simulink model "aerotest"  (R2021b)
settings: Solver=VariableStepAuto  StartTime=0.0  StopTime=10.0  RelTol=1e-3
undefined symbols (not defined in the file or in its folder): admireDB
libraries: simulink_extras x103, simulink x24, aerolibatmos2 x1
(part 5 of 13)

== system aerotest/RollMomentCoefficient/MachRegion1/Crmbetad ==
  in_bus : Inport
  Bus Selector : BusSelector  OutputSignals=AeroIn_Bus.angleOfAttack_deg,AeroIn_Bus.betad
  Crmbetad_ : Subsystem
  Crmbetad : Outport
  wires:
  Bus Selector/1 -> Crmbetad_/1(angleOfAttack_deg)  "<angleOfAttack_deg>"
  Bus Selector/2 -> Crmbetad_/2(betad)  "<betad>"
  in_bus/1 -> Bus Selector/1  "in_bus"
  Crmbetad_/1(Crmbetad) -> Crmbetad/1

== system aerotest/RollMomentCoefficient/MachRegion1/Crmblg ==
  in_bus : Inport
  Bus Selector : BusSelector  OutputSignals=AeroIn_Bus.lg_bool,AeroIn_Bus.angleOfAttack_deg,AeroIn_Bus.angleOfSideslip_deg
  Crmblg_ : Subsystem
  Crmblg : Outport
  wires:
  Bus Selector/3 -> Crmblg_/3(angleOfSideslip_deg)  "<angleOfSideslip_deg>"
  Bus Selector/2 -> Crmblg_/2(angleOfAttack_deg)  "<angleOfAttack_deg>"
  Bus Selector/1 -> Crmblg_/1(dLG)  "<lg_bool>"
  in_bus/1 -> Bus Selector/1  "in_bus"
  Crmblg_/1(Crmblg) -> Crmblg/1

== system aerotest/RollMomentCoefficient/MachRegion1/Crmdai ==
  in_bus : Inport
  Bus Selector : BusSelector  OutputSignals=AeroIn_Bus.dAI,AeroIn_Bus.angleOfAttack_deg,AeroIn_Bus.dEI,eieff,AeroIn_Bus.qacorr,AeroIn_Bus.mach_nd
  Crmdai_ : Subsystem
  Crmdai : Outport
  wires:
  Bus Selector/1 -> Crmdai_/1(dAI)  "<dAI>"
  Bus Selector/2 -> Crmdai_/2(angleOfAttack_deg)  "<angleOfAttack_deg>"
  Bus Selector/3 -> Crmdai_/3(dEI)  "<dEI>"
  Bus Selector/4 -> Crmdai_/4(eieff)  "<eieff>"
  Bus Selector/5 -> Crmdai_/5(qacorr)  "<qacorr>"
  Bus Selector/6 -> Crmdai_/6(mach_nd)  "<mach_nd>"
  in_bus/1 -> Bus Selector/1  "in_bus"
  Crmdai_/1(Crmdai) -> Crmdai/1

== system aerotest/RollMomentCoefficient/MachRegion1/Crmdaib ==
  in_bus : Inport
  Bus Selector : BusSelector  OutputSignals=AeroIn_Bus.angleOfAttack_deg,AeroIn_Bus.dAI,AeroIn_Bus.angleOfSideslip_deg,eieff
  Crmdaib_ : Subsystem
  Crmdaib : Outport
  wires:
  Bus Selector/1 -> Crmdaib_/1(angleOfAttack_deg)  "<angleOfAttack_deg>"
  Bus Selector/2 -> Crmdaib_/2(dAI)  "<dAI>"
  Bus Selector/3 -> Crmdaib_/3(angleOfSideslip_deg)  "<angleOfSideslip_deg>"
  Bus Selector/4 -> Crmdaib_/4(eieff)  "<eieff>"
  Crmdaib_/1(Crmdaib) -> Crmdaib/1
  in_bus/1 -> Bus Selector/1  "in_bus"

== system aerotest/RollMomentCoefficient/MachRegion1/Crmday ==
  in_bus : Inport
  Bus Selector : BusSelector  OutputSignals=AeroIn_Bus.dAY,AeroIn_Bus.angleOfAttack_deg,AeroIn_Bus.dEY,eoeff,AeroIn_Bus.qacorr,AeroIn_Bus.mach_nd
  Crmday_ : Subsystem
  Crmday : Outport
  wires:
  Crmday_/1(Crmdai) -> Crmday/1
  in_bus/1 -> Bus Selector/1  "in_bus"
  Bus Selector/6 -> Crmday_/6(mach_nd)  "<mach_nd>"
  Bus Selector/5 -> Crmday_/5(qacorr)  "<qacorr>"
  Bus Selector/4 -> Crmday_/4(eoeff)  "<eoeff>"
  Bus Selector/3 -> Crmday_/3(dEY)  "<dEY>"
  Bus Selector/2 -> Crmday_/2(angleOfAttack_deg)  "<angleOfAttack_deg>"
  Bus Selector/1 -> Crmday_/1(dAY)  "<dAY>"

== system aerotest/RollMomentCoefficient/MachRegion1/Crmdayb ==
  in_bus : Inport
  Bus Selector : BusSelector  OutputSignals=AeroIn_Bus.angleOfAttack_deg,AeroIn_Bus.dAY,AeroIn_Bus.angleOfSideslip_deg,eoeff
  Crmdaib_ : Subsystem
  Crmdayb : Outport
  wires:
  in_bus/1 -> Bus Selector/1  "in_bus"
  Crmdaib_/1(Crmdaib) -> Crmdayb/1
  Bus Selector/4 -> Crmdaib_/4(eoeff)  "<eoeff>"
  Bus Selector/3 -> Crmdaib_/3(angleOfSideslip_deg)  "<angleOfSideslip_deg>"
  Bus Selector/2 -> Crmdaib_/2(dAY)  "<dAY>"
  Bus Selector/1 -> Crmdaib_/1(angleOfAttack_deg)  "<angleOfAttack_deg>"

== system aerotest/RollMomentCoefficient/MachRegion1/Crmdna ==
  in_bus : Inport
  Bus Selector : BusSelector  OutputSignals=AeroIn_Bus.dNE,AeroIn_Bus.angleOfAttack_deg,AeroIn_Bus.dNA
  Crmdna_ : Subsystem
  Crmdna : Outport
  wires:
  Bus Selector/3 -> Crmdna_/3(dNA)  "<dNA>"
  Bus Selector/2 -> Crmdna_/2(angleOfAttack_deg)  "<angleOfAttack_deg>"
  Bus Selector/1 -> Crmdna_/1(dNE)  "<dNE>"
  Crmdna_/1(Crmdna) -> Crmdna/1
  in_bus/1 -> Bus Selector/1  "in_bus"

== system aerotest/RollMomentCoefficient/MachRegion1/Crmdr ==
  in_bus : Inport
  Bus Selector : BusSelector  OutputSignals=AeroIn_Bus.angleOfAttack_deg,AeroIn_Bus.rud_deg,AeroIn_Bus.angleOfSideslip_deg,AeroIn_Bus.qacorr,AeroIn_Bus.mach_nd
  Crmdr_ : Subsystem
  Crmdr : Outport
  wires:
  Bus Selector/5 -> Crmdr_/5(mach_nd)  "<mach_nd>"
  Bus Selector/4 -> Crmdr_/4(qacorr)  "<qacorr>"
  Bus Selector/3 -> Crmdr_/3(angleOfSideslip_deg)  "<angleOfSideslip_deg>"
  Bus Selector/2 -> Crmdr_/2(dR)  "<rud_deg>"
  Bus Selector/1 -> Crmdr_/1(angleOfAttack_deg)  "<angleOfAttack_deg>"
  Crmdr_/1(Crmdr) -> Crmdr/1
  in_bus/1 -> Bus Selector/1  "in_bus"

== system aerotest/RollMomentCoefficient/MachRegion1/Crmp ==
  in_bus : Inport
  Bus Selector : BusSelector  OutputSignals=AeroIn_Bus.dN,AeroIn_Bus.angleOfAttack_deg,AeroIn_Bus.qacorr,AeroIn_Bus.mach_nd,AeroIn_Bus.pc
  Crmp_ : Subsystem
  Crmp : Outport
  wires:
  Bus Selector/1 -> Crmp_/1(dN)  "<dN>"
  Bus Selector/2 -> Crmp_/2(angleOfAttack_deg)  "<angleOfAttack_deg>"
  Bus Selector/3 -> Crmp_/3(qacorr)  "<qacorr>"
  Bus Selector/4 -> Crmp_/4(mach_nd)  "<mach_nd>"
  Bus Selector/5 -> Crmp_/5(pc)  "<pc>"
  Crmp_/1(Crmp) -> Crmp/1
  in_bus/1 -> Bus Selector/1  "in_bus"

== system aerotest/RollMomentCoefficient/MachRegion1/Crmpbeta ==
  in_bus : Inport
  Bus Selector : BusSelector  OutputSignals=AeroIn_Bus.angleOfSideslip_deg,AeroIn_Bus.angleOfAttack_deg,AeroIn_Bus.pc
  Crmpbeta_ : Subsystem
  Crmpbeta : Outport
  wires:
  Bus Selector/1 -> Crmpbeta_/1(angleOfSideslip_deg)  "<angleOfSideslip_deg>"
  Bus Selector/2 -> Crmpbeta_/2(angleOfAttack_deg)  "<angleOfAttack_deg>"
  Bus Selector/3 -> Crmpbeta_/3(pc)  "<pc>"
  in_bus/1 -> Bus Selector/1  "in_bus"
  Crmpbeta_/1(Crmpbeta) -> Crmpbeta/1

== system aerotest/RollMomentCoefficient/MachRegion1/Crmr ==
  in_bus : Inport
  Bus Selector : BusSelector  OutputSignals=AeroIn_Bus.dN,AeroIn_Bus.angleOfAttack_deg,AeroIn_Bus.rc
  Crmr_ : Subsystem
  Crmr : Outport
  wires:
  Bus Selector/1 -> Crmr_/1(dN)  "<dN>"
  Bus Selector/2 -> Crmr_/2(angleOfAttack_deg)  "<angleOfAttack_deg>"
  Bus Selector/3 -> Crmr_/3(rc)  "<rc>"
  Crmr_/1(Crmr) -> Crmr/1
  in_bus/1 -> Bus Selector/1  "in_bus"

== system aerotest/RollMomentCoefficient/MachRegion1/Crmrbeta ==
  in_bus : Inport
  Bus Selector : BusSelector  OutputSignals=AeroIn_Bus.angleOfSideslip_deg,AeroIn_Bus.angleOfAttack_deg,AeroIn_Bus.rc
  Crmrbeta_ : Subsystem
  Crmrbeta : Outport
  wires:
  in_bus/1 -> Bus Selector/1  "in_bus"
  Crmrbeta_/1(Crmrbeta) -> Crmrbeta/1
  Bus Selector/3 -> Crmrbeta_/3(rc)  "<rc>"
  Bus Selector/2 -> Crmrbeta_/2(angleOfAttack_deg)  "<angleOfAttack_deg>"
  Bus Selector/1 -> Crmrbeta_/1(angleOfSideslip_deg)  "<angleOfSideslip_deg>"

== system aerotest/RollMomentCoefficient/MachRegion1/Crmrde ==
  in_bus : Inport
  Bus Selector : BusSelector  OutputSignals=AeroIn_Bus.mach_nd,AeroIn_Bus.angleOfAttack_deg,AeroIn_Bus.rc,AeroIn_Bus.dEI,eieff,AeroIn_Bus.dEY,eoeff
  Crmrde_ : Subsystem
  Crmrbeta : Outport
  wires:
  Bus Selector/1 -> Crmrde_/1(mach_nd)  "<mach_nd>"
  Bus Selector/2 -> Crmrde_/2(angleOfAttack_deg)  "<angleOfAttack_deg>"
  Bus Selector/3 -> Crmrde_/3(rc)  "<rc>"
  Bus Selector/4 -> Crmrde_/4(dEI)  "<dEI>"
  Bus Selector/5 -> Crmrde_/5(eieff)  "<eieff>"
  Bus Selector/6 -> Crmrde_/6(dey)  "<dEY>"
  Bus Selector/7 -> Crmrde_/7(eoeff)  "<eoeff>"
  Crmrde_/1(Crmrbeta) -> Crmrbeta/1
  in_bus/1 -> Bus Selector/1  "in_bus"

== system aerotest/RollMomentCoefficient/MachRegion1/eoeff1 ==
  AeroIn_Bus : Inport
  Bus Selector : BusSelector  OutputSignals=mach_nd
  CRMDAYOD_M : Lookup_n-D  NumberOfTableDimensions=1  BreakpointsForDimension1=admireDB.aerodata_asym_ext.CRMDAYOD.breakpoints.M  BreakpointsForDimension3=[5, 7]  Table=admireDB.aerodata_asym_ext.CRMDAYOD.newTable  ExtrapMethod=Clip  InternalRulePriority=Speed  RndMeth=Simplest  InputSameDT=on
  Constant : Constant
  Sum : Sum  Inputs=-+|
  eoeff : Outport
  eieff : Outport  Port=2
  wires:
  Sum/1 -> eieff/1
  CRMDAYOD_M/1 -> eoeff/1, Sum/1
  Constant/1 -> Sum/2
  Bus Selector/1 -> CRMDAYOD_M/1  "<mach_nd>"
  AeroIn_Bus/1 -> Bus Selector/1

== system aerotest/RollMomentCoefficient/MachRegion2/Crmbasic ==
  in_bus : Inport
  Bus Selector : BusSelector  OutputSignals=AeroIn_Bus.angleOfAttack_deg,AeroIn_Bus.tflow
  Crmbasic_ : Subsystem
  Crmbasic : Outport
  wires:
  Bus Selector/2 -> Crmbasic_/2(tflow)  "<tflow>"
  Crmbasic_/1(Crmbasic) -> Crmbasic/1
  Bus Selector/1 -> Crmbasic_/1(angleOfAttack_deg)  "<angleOfAttack_deg>"
  in_bus/1 -> Bus Selector/1  "in_bus"

== system aerotest/RollMomentCoefficient/MachRegion2/Crmbde ==
  in_bus : Inport
  Bus Selector : BusSelector  OutputSignals=AeroIn_Bus.angleOfAttack_deg,AeroIn_Bus.dN,AeroIn_Bus.dEI,AeroIn_Bus.angleOfSideslip_deg,AeroIn_Bus.dEY,eieff,eoeff
  Crmbde_ : Subsystem
  Crmbde : Outport
  wires:
  Bus Selector/1 -> Crmbde_/1(angleOfAttack_deg)  "<angleOfAttack_deg>"
  Bus Selector/2 -> Crmbde_/2(dN)  "<dN>"
  Bus Selector/3 -> Crmbde_/3(dEI)  "<dEI>"
  Bus Selector/4 -> Crmbde_/4(angleOfSideslip_deg)  "<angleOfSideslip_deg>"
  Bus Selector/5 -> Crmbde_/5(dEY)  "<dEY>"
  Bus Selector/6 -> Crmbde_/6(eieff)  "<eieff>"
  Bus Selector/7 -> Crmbde_/7(eoeff)  "<eoeff>"
  Crmbde_/1(Crmbde) -> Crmbde/1
  in_bus/1 -> Bus Selector/1  "in_bus"

== system aerotest/RollMomentCoefficient/MachRegion2/Crmbdle ==
  in_bus : Inport
  Bus Selector : BusSelector  OutputSignals=AeroIn_Bus.angleOfAttack_deg,AeroIn_Bus.dEI,AeroIn_Bus.angleOfSideslip_deg,AeroIn_Bus.lef_deg,AeroIn_Bus.dEY,AeroIn_Bus.tflow,AeroIn_Bus.tfhigh
  Crmbdle_ : Subsystem
  Crmbdle : Outport
  wires:
  Bus Selector/7 -> Crmbdle_/7(tfhigh)  "<tfhigh>"
  Bus Selector/6 -> Crmbdle_/6(tflow)  "<tflow>"
  Bus Selector/5 -> Crmbdle_/5(dEY)  "<dEY>"
  Bus Selector/4 -> Crmbdle_/4(dLE)  "<lef_deg>"
  Bus Selector/3 -> Crmbdle_/3(angleOfSideslip_deg)  "<angleOfSideslip_deg>"
  Bus Selector/2 -> Crmbdle_/2(dEI)  "<dEI>"
  Bus Selector/1 -> Crmbdle_/1(angleOfAttack_deg)  "<angleOfAttack_deg>"
  Crmbdle_/1(Crmbdle) -> Crmbdle/1
  in_bus/1 -> Bus Selector/1  "in_bus"

== system aerotest/RollMomentCoefficient/MachRegion2/Crmbdn ==
  in_bus : Inport
  Bus Selector : BusSelector  OutputSignals=AeroIn_Bus.angleOfSideslip_deg,AeroIn_Bus.dN,AeroIn_Bus.angleOfAttack_deg,AeroIn_Bus.tflow,AeroIn_Bus.tfhigh
  Crmbdn_ : Subsystem
  Crmbdn : Outport
  wires:
  Bus Selector/1 -> Crmbdn_/1(angleOfSideslip_deg)  "<angleOfSideslip_deg>"
  Bus Selector/2 -> Crmbdn_/2(dN)  "<dN>"
  Bus Selector/3 -> Crmbdn_/3(angleOfAttack_deg)  "<angleOfAttack_deg>"
  Bus Selector/4 -> Crmbdn_/4(tflow)  "<tflow>"
  Bus Selector/5 -> Crmbdn_/5(tfhigh)  "<tfhigh>"
  in_bus/1 -> Bus Selector/1  "in_bus"
  Crmbdn_/1(Crmbdn) -> Crmbdn/1

== system aerotest/RollMomentCoefficient/MachRegion2/Crmbeta ==
  in_bus : Inport
  Bus Selector : BusSelector  OutputSignals=AeroIn_Bus.angleOfSideslip_deg,AeroIn_Bus.angleOfAttack_deg,AeroIn_Bus.tflow,AeroIn_Bus.tfhigh,AeroIn_Bus.qacorr,AeroIn_Bus.mach_nd
  Crmbeta_ : Subsystem
  Crmbeta : Outport
  wires:
  Bus Selector/1 -> Crmbeta_/1(angleOfSideslip_deg)  "<angleOfSideslip_deg>"
  Bus Selector/2 -> Crmbeta_/2(angleOfAttack_deg)  "<angleOfAttack_deg>"
  Bus Selector/3 -> Crmbeta_/3(tflow)  "<tflow>"
  Bus Selector/4 -> Crmbeta_/4(thigh)  "<tfhigh>"
  Bus Selector/5 -> Crmbeta_/5(qacorr)  "<qacorr>"
  Bus Selector/6 -> Crmbeta_/6(mach_nd)  "<mach_nd>"
  in_bus/1 -> Bus Selector/1  "in_bus"
  Crmbeta_/1(Crmbeta) -> Crmbeta/1

== system aerotest/RollMomentCoefficient/MachRegion2/Crmbetad ==
  in_bus : Inport
  Bus Selector : BusSelector  OutputSignals=AeroIn_Bus.angleOfAttack_deg,AeroIn_Bus.betad,AeroIn_Bus.tflow,AeroIn_Bus.tfhigh
  Crmbetad_ : Subsystem
  Crmbetad : Outport
  wires:
  Bus Selector/1 -> Crmbetad_/1(angleOfAttack_deg)  "<angleOfAttack_deg>"
  Bus Selector/2 -> Crmbetad_/2(betad)  "<betad>"
  Bus Selector/3 -> Crmbetad_/3(tflow)  "<tflow>"
  Bus Selector/4 -> Crmbetad_/4(tfhigh)  "<tfhigh>"
  in_bus/1 -> Bus Selector/1  "in_bus"
  Crmbetad_/1(Crmbetad) -> Crmbetad/1

== system aerotest/RollMomentCoefficient/MachRegion2/Crmblg ==
  in_bus : Inport
  Bus Selector : BusSelector  OutputSignals=AeroIn_Bus.lg_bool,AeroIn_Bus.angleOfAttack_deg,AeroIn_Bus.angleOfSideslip_deg
  Crmblg_ : Subsystem
  Crmblg : Outport
  wires:
  Bus Selector/3 -> Crmblg_/3(angleOfSideslip_deg)  "<angleOfSideslip_deg>"
  Bus Selector/2 -> Crmblg_/2(angleOfAttack_deg)  "<angleOfAttack_deg>"
  Bus Selector/1 -> Crmblg_/1(dLG)  "<lg_bool>"
  in_bus/1 -> Bus Selector/1  "in_bus"
  Crmblg_/1(Crmblg) -> Crmblg/1

== system aerotest/RollMomentCoefficient/MachRegion2/Crmdai ==
  in_bus : Inport
  Bus Selector : BusSelector  OutputSignals=AeroIn_Bus.dAI,AeroIn_Bus.angleOfAttack_deg,AeroIn_Bus.dEI,eieff,AeroIn_Bus.qacorr,AeroIn_Bus.mach_nd,AeroIn_Bus.tflow,AeroIn_Bus.tfhigh
  Crmdai_ : Subsystem
  Crmdai : Outport
  wires:
  Bus Selector/8 -> Crmdai_/8(tfhigh)  "<tfhigh>"
  Bus Selector/7 -> Crmdai_/7(tflow)  "<tflow>"
  Bus Selector/6 -> Crmdai_/6(mach_nd)  "<mach_nd>"
  Bus Selector/5 -> Crmdai_/5(qacorr)  "<qacorr>"
  Bus Selector/4 -> Crmdai_/4(eieff)  "<eieff>"
  Bus Selector/3 -> Crmdai_/3(dEI)  "<dEI>"
  Bus Selector/2 -> Crmdai_/2(angleOfAttack_deg)  "<angleOfAttack_deg>"
  Bus Selector/1 -> Crmdai_/1(dAI)  "<dAI>"
  in_bus/1 -> Bus Selector/1  "in_bus"
  Crmdai_/1(Crmdai) -> Crmdai/1

== system aerotest/RollMomentCoefficient/MachRegion2/Crmdaib ==
  in_bus : Inport
  Bus Selector : BusSelector  OutputSignals=AeroIn_Bus.angleOfAttack_deg,AeroIn_Bus.dAI,AeroIn_Bus.angleOfSideslip_deg,eieff,AeroIn_Bus.tflow
  Crmdaib_ : Subsystem
  Crmdaib : Outport
  wires:
  Bus Selector/1 -> Crmdaib_/1(angleOfAttack_deg)  "<angleOfAttack_deg>"
  Bus Selector/2 -> Crmdaib_/2(dAI)  "<dAI>"
  Bus Selector/3 -> Crmdaib_/3(angleOfSideslip_deg)  "<angleOfSideslip_deg>"
  Bus Selector/4 -> Crmdaib_/4(eieff)  "<eieff>"
  Bus Selector/5 -> Crmdaib_/5(tflow)  "<tflow>"
  Crmdaib_/1(Crmdaib) -> Crmdaib/1
  in_bus/1 -> Bus Selector/1  "in_bus"

== system aerotest/RollMomentCoefficient/MachRegion2/Crmday ==
  in_bus : Inport
  Bus Selector : BusSelector  OutputSignals=AeroIn_Bus.dAY,AeroIn_Bus.angleOfAttack_deg,AeroIn_Bus.dEY,eoeff,AeroIn_Bus.qacorr,AeroIn_Bus.mach_nd,AeroIn_Bus.tflow,AeroIn_Bus.tfhigh
  Crmday_ : Subsystem
  Crmday : Outport
  wires:
  Bus Selector/8 -> Crmday_/8(tfhigh)  "<tfhigh>"
  Bus Selector/7 -> Crmday_/7(tflow)  "<tflow>"
  Bus Selector/6 -> Crmday_/6(mach_nd)  "<mach_nd>"
  Bus Selector/5 -> Crmday_/5(qacorr)  "<qacorr>"
  Bus Selector/4 -> Crmday_/4(eoeff)  "<eoeff>"
  Bus Selector/3 -> Crmday_/3(dEY)  "<dEY>"
  Bus Selector/2 -> Crmday_/2(angleOfAttack_deg)  "<angleOfAttack_deg>"
  Bus Selector/1 -> Crmday_/1(dAY)  "<dAY>"
  Crmday_/1(Crmdai) -> Crmday/1
  in_bus/1 -> Bus Selector/1  "in_bus"

== system aerotest/RollMomentCoefficient/MachRegion2/Crmdayb ==
  in_bus : Inport
  Bus Selector : BusSelector  OutputSignals=AeroIn_Bus.angleOfAttack_deg,AeroIn_Bus.dAY,AeroIn_Bus.angleOfSideslip_deg,eoeff,AeroIn_Bus.tflow
  Crmdayb_ : Subsystem
  Crmdayb : Outport
  wires:
  Bus Selector/5 -> Crmdayb_/5(tflow)  "<tflow>"
  Bus Selector/4 -> Crmdayb_/4(eoeff)  "<eoeff>"
  Bus Selector/3 -> Crmdayb_/3(angleOfSideslip_deg)  "<angleOfSideslip_deg>"
  Bus Selector/2 -> Crmdayb_/2(dAY)  "<dAY>"
  Bus Selector/1 -> Crmdayb_/1(angleOfAttack_deg)  "<angleOfAttack_deg>"
  in_bus/1 -> Bus Selector/1  "in_bus"
  Crmdayb_/1(Crmdayb) -> Crmdayb/1

== system aerotest/RollMomentCoefficient/MachRegion2/Crmdna ==
  in_bus : Inport
  Bus Selector : BusSelector  OutputSignals=AeroIn_Bus.dNE,AeroIn_Bus.angleOfAttack_deg,AeroIn_Bus.tflow,AeroIn_Bus.tfhigh,AeroIn_Bus.dNA
  Crmdna_ : Subsystem
  Crmdna : Outport
  wires:
  Bus Selector/1 -> Crmdna_/1(dNE)  "<dNE>"
  Bus Selector/2 -> Crmdna_/2(angleOfAttack_deg)  "<angleOfAttack_deg>"
  Bus Selector/3 -> Crmdna_/3(tflow)  "<tflow>"
  Bus Selector/4 -> Crmdna_/4(tfhigh)  "<tfhigh>"
  Bus Selector/5 -> Crmdna_/5(dNA)  "<dNA>"
  Crmdna_/1(Crmdna) -> Crmdna/1
  in_bus/1 -> Bus Selector/1  "in_bus"

== system aerotest/RollMomentCoefficient/MachRegion2/Crmdr ==
  in_bus : Inport
  Bus Selector : BusSelector  OutputSignals=AeroIn_Bus.angleOfAttack_deg,AeroIn_Bus.rud_deg,AeroIn_Bus.tfhigh,AeroIn_Bus.angleOfSideslip_deg,AeroIn_Bus.tflow,AeroIn_Bus.qacorr,AeroIn_Bus.mach_nd
  Crmdr_ : Subsystem
  Crmdr : Outport
  wires:
  Bus Selector/1 -> Crmdr_/1(angleOfAttack_deg)  "<angleOfAttack_deg>"
  Bus Selector/2 -> Crmdr_/2(dR)  "<rud_deg>"
  Bus Selector/7 -> Crmdr_/7(mach_nd)  "<mach_nd>"
  Bus Selector/3 -> Crmdr_/3(tfhigh)  "<tfhigh>"
  Bus Selector/6 -> Crmdr_/6(qacorr)  "<qacorr>"
  Bus Selector/4 -> Crmdr_/4(angleOfSideslip_deg)  "<angleOfSideslip_deg>"
  Bus Selector/5 -> Crmdr_/5(tflow)  "<tflow>"
  Crmdr_/1(Crmdr) -> Crmdr/1
  in_bus/1 -> Bus Selector/1  "in_bus"

== system aerotest/RollMomentCoefficient/MachRegion2/Crmp ==
  in_bus : Inport
  Bus Selector : BusSelector  OutputSignals=AeroIn_Bus.dN,AeroIn_Bus.angleOfAttack_deg,AeroIn_Bus.qacorr,AeroIn_Bus.mach_nd,AeroIn_Bus.pc,AeroIn_Bus.tflow,AeroIn_Bus.tfhigh
  Crmp_ : Subsystem
  Crmp : Outport
  wires:
  Bus Selector/7 -> Crmp_/7(tfhigh)  "<tfhigh>"
  Bus Selector/1 -> Crmp_/1(dN)  "<dN>"
  Bus Selector/6 -> Crmp_/6(tflow)  "<tflow>"
  Bus Selector/2 -> Crmp_/2(angleOfAttack_deg)  "<angleOfAttack_deg>"
  Bus Selector/5 -> Crmp_/5(pc)  "<pc>"
  Bus Selector/3 -> Crmp_/3(qacorr)  "<qacorr>"
  Bus Selector/4 -> Crmp_/4(mach_nd)  "<mach_nd>"
  Crmp_/1(Crmp) -> Crmp/1
  in_bus/1 -> Bus Selector/1  "in_bus"

== system aerotest/RollMomentCoefficient/MachRegion2/Crmpbeta ==
  in_bus : Inport
  Bus Selector : BusSelector  OutputSignals=AeroIn_Bus.angleOfSideslip_deg,AeroIn_Bus.pc,AeroIn_Bus.angleOfAttack_deg,AeroIn_Bus.tflow
  Crmpbeta_ : Subsystem
  Crmpbeta : Outport
  wires:
  Bus Selector/4 -> Crmpbeta_/4(tflow)  "<tflow>"
  Bus Selector/3 -> Crmpbeta_/3(angleOfAttack_deg)  "<angleOfAttack_deg>"
  Bus Selector/1 -> Crmpbeta_/1(angleOfSideslip_deg)  "<angleOfSideslip_deg>"
  Bus Selector/2 -> Crmpbeta_/2(pc)  "<pc>"
  in_bus/1 -> Bus Selector/1  "in_bus"
  Crmpbeta_/1(Crmpbeta) -> Crmpbeta/1

== system aerotest/RollMomentCoefficient/MachRegion2/Crmr ==
  in_bus : Inport
  Bus Selector : BusSelector  OutputSignals=AeroIn_Bus.dN,AeroIn_Bus.angleOfAttack_deg,AeroIn_Bus.rc,AeroIn_Bus.tflow,AeroIn_Bus.tfhigh
  Crmr_ : Subsystem
  Crmr : Outport
  wires:
  Bus Selector/5 -> Crmr_/5(tfhigh)  "<tfhigh>"
  Bus Selector/4 -> Crmr_/4(tflow)  "<tflow>"
  Bus Selector/3 -> Crmr_/3(rc)  "<rc>"
  Bus Selector/2 -> Crmr_/2(angleOfAttack_deg)  "<angleOfAttack_deg>"
  Bus Selector/1 -> Crmr_/1(dN)  "<dN>"
  Crmr_/1(Crmr) -> Crmr/1
  in_bus/1 -> Bus Selector/1  "in_bus"

== system aerotest/RollMomentCoefficient/MachRegion2/Crmrbeta ==
  in_bus : Inport
  Bus Selector : BusSelector  OutputSignals=AeroIn_Bus.angleOfSideslip_deg,AeroIn_Bus.angleOfAttack_deg,AeroIn_Bus.rc,AeroIn_Bus.tflow
  Crmrbeta_ : Subsystem
  Crmrbeta : Outport
  wires:
  Bus Selector/1 -> Crmrbeta_/1(angleOfSideslip_deg)  "<angleOfSideslip_deg>"
  Bus Selector/2 -> Crmrbeta_/2(angleOfAttack_deg)  "<angleOfAttack_deg>"
  Bus Selector/3 -> Crmrbeta_/3(rc)  "<rc>"
  Bus Selector/4 -> Crmrbeta_/4(tflow)  "<tflow>"
  in_bus/1 -> Bus Selector/1  "in_bus"
  Crmrbeta_/1(Crmrbeta) -> Crmrbeta/1

== system aerotest/RollMomentCoefficient/MachRegion2/Crmrde ==
  in_bus : Inport
  Bus Selector : BusSelector  OutputSignals=AeroIn_Bus.mach_nd,AeroIn_Bus.angleOfAttack_deg,AeroIn_Bus.rc,AeroIn_Bus.dEI,eieff,AeroIn_Bus.dEY,eoeff
  Crmrde_ : Subsystem
  Crmrde : Outport
  wires:
  Bus Selector/7 -> Crmrde_/7(eoeff)  "<eoeff>"
  Bus Selector/1 -> Crmrde_/1(mach_nd)  "<mach_nd>"
  Bus Selector/6 -> Crmrde_/6(dey)  "<dEY>"
  Bus Selector/2 -> Crmrde_/2(angleOfAttack_deg)  "<angleOfAttack_deg>"
  Bus Selector/5 -> Crmrde_/5(eieff)  "<eieff>"
  Bus Selector/3 -> Crmrde_/3(rc)  "<rc>"
  Bus Selector/4 -> Crmrde_/4(dEI)  "<dEI>"
  Crmrde_/1(Crmrde) -> Crmrde/1
  in_bus/1 -> Bus Selector/1  "in_bus"

== system aerotest/RollMomentCoefficient/MachRegion2/eoeff1 ==
  AeroIn_Bus : Inport
  Bus Selector : BusSelector  OutputSignals=mach_nd
  CRMDAYOD_M : Lookup_n-D  NumberOfTableDimensions=1  BreakpointsForDimension1=admireDB.aerodata_asym_ext.CRMDAYOD.breakpoints.M  BreakpointsForDimension3=[5, 7]  Table=admireDB.aerodata_asym_ext.CRMDAYOD.newTable  ExtrapMethod=Clip  InternalRulePriority=Speed  RndMeth=Simplest  InputSameDT=on
  Constant : Constant
  Sum : Sum  Inputs=-+|
  eoeff : Outport
  eieff : Outport  Port=2
  wires:
  Sum/1 -> eieff/1
  CRMDAYOD_M/1 -> eoeff/1, Sum/1
  Constant/1 -> Sum/2
  Bus Selector/1 -> CRMDAYOD_M/1  "<mach_nd>"
  AeroIn_Bus/1 -> Bus Selector/1

== system aerotest/RollMomentCoefficient/MachRegion3/Crmbasic ==
  Constant : Constant  Value=0
  Crmbasic : Outport
  wires:
  Constant/1 -> Crmbasic/1

== system aerotest/RollMomentCoefficient/MachRegion3/Crmbde ==
  in_bus : Inport
  Bus Selector : BusSelector  OutputSignals=AeroIn_Bus.angleOfAttack_deg,AeroIn_Bus.dN,AeroIn_Bus.dEI,AeroIn_Bus.angleOfSideslip_deg,AeroIn_Bus.dEY,eieff,eoeff,AeroIn_Bus.mach_nd
  Crmbde_ : Subsystem
  Crmbde : Outport
  wires:
  Bus Selector/8 -> Crmbde_/8(mach_nd)  "<mach_nd>"
  Bus Selector/7 -> Crmbde_/7(eoeff)  "<eoeff>"
  Bus Selector/6 -> Crmbde_/6(eieff)  "<eieff>"
  Bus Selector/5 -> Crmbde_/5(dEY)  "<dEY>"
  Bus Selector/4 -> Crmbde_/4(angleOfSideslip_deg)  "<angleOfSideslip_deg>"
  Bus Selector/3 -> Crmbde_/3(dEI)  "<dEI>"
  Bus Selector/2 -> Crmbde_/2(dN)  "<dN>"
  Bus Selector/1 -> Crmbde_/1(angleOfAttack_deg)  "<angleOfAttack_deg>"
  Crmbde_/1(Crmbde) -> Crmbde/1
  in_bus/1 -> Bus Selector/1  "in_bus"

== system aerotest/RollMomentCoefficient/MachRegion3/Crmbdle ==
  in_bus : Inport
  Bus Selector : BusSelector  OutputSignals=AeroIn_Bus.angleOfAttack_deg,AeroIn_Bus.dEI,AeroIn_Bus.mach_nd,AeroIn_Bus.dEY,eieff,eoeff,AeroIn_Bus.angleOfSideslip_deg,AeroIn_Bus.lef_deg
  Crmbdle_ : Subsystem
  Crmbdle : Outport
  wires:
  Bus Selector/1 -> Crmbdle_/1(angleOfAttack_deg)  "<angleOfAttack_deg>"
  Bus Selector/2 -> Crmbdle_/2(dEI)  "<dEI>"
  Bus Selector/3 -> Crmbdle_/3(mach_nd)  "<mach_nd>"
  Bus Selector/4 -> Crmbdle_/4(dEY)  "<dEY>"
  Bus Selector/5 -> Crmbdle_/5(eieff)  "<eieff>"
  Bus Selector/6 -> Crmbdle_/6(eoeff)  "<eoeff>"
  Bus Selector/7 -> Crmbdle_/7(angleOfSideslip_deg)  "<angleOfSideslip_deg>"
  Bus Selector/8 -> Crmbdle_/8(dLE)  "<lef_deg>"
  Crmbdle_/1(Crmbdle) -> Crmbdle/1
  in_bus/1 -> Bus Selector/1  "in_bus"

== system aerotest/RollMomentCoefficient/MachRegion3/Crmbdn ==
  in_bus : Inport
  Bus Selector : BusSelector  OutputSignals=AeroIn_Bus.dN,AeroIn_Bus.mach_nd,AeroIn_Bus.angleOfSideslip_deg
  Crmbdn_ : Subsystem
  Crmbdn : Outport
  wires:
  Bus Selector/3 -> Crmbdn_/3(angleOfSideslip_deg)  "<angleOfSideslip_deg>"
  Bus Selector/1 -> Crmbdn_/1(dN)  "<dN>"
  Bus Selector/2 -> Crmbdn_/2(mach_nd)  "<mach_nd>"
  in_bus/1 -> Bus Selector/1  "in_bus"
  Crmbdn_/1(Crmbdn) -> Crmbdn/1

== system aerotest/RollMomentCoefficient/MachRegion3/Crmbeta ==
  in_bus : Inport
  Bus Selector : BusSelector  OutputSignals=AeroIn_Bus.mach_nd,AeroIn_Bus.angleOfAttack_deg,AeroIn_Bus.angleOfSideslip_deg,AeroIn_Bus.qacorr
  Crmbeta_ : Subsystem
  Crmbeta : Outport
  wires:
  Bus Selector/2 -> Crmbeta_/2(angleOfAttack_deg)  "<angleOfAttack_deg>"
  Bus Selector/1 -> Crmbeta_/1(mach_nd)  "<mach_nd>"
  Bus Selector/3 -> Crmbeta_/3(angleOfSideslip_deg)  "<angleOfSideslip_deg>"
  Bus Selector/4 -> Crmbeta_/4(qacorr)  "<qacorr>"
  in_bus/1 -> Bus Selector/1  "in_bus"
  Crmbeta_/1(Crmbeta) -> Crmbeta/1

== system aerotest/RollMomentCoefficient/MachRegion3/Crmbetad ==
  in_bus : Inport
  Bus Selector : BusSelector  OutputSignals=AeroIn_Bus.angleOfAttack_deg,AeroIn_Bus.mach_nd,AeroIn_Bus.betad
  Crmbetad_ : Subsystem
  Crmbetad : Outport
  wires:
  Bus Selector/3 -> Crmbetad_/3(betad)  "<betad>"
  Bus Selector/1 -> Crmbetad_/1(angleOfAttack_deg)  "<angleOfAttack_deg>"
  Bus Selector/2 -> Crmbetad_/2(mach_nd)  "<mach_nd>"
  in_bus/1 -> Bus Selector/1  "in_bus"
  Crmbetad_/1(Crmbetad) -> Crmbetad/1

== system aerotest/RollMomentCoefficient/MachRegion3/Crmblg ==
  in_bus : Inport
  Bus Selector : BusSelector  OutputSignals=AeroIn_Bus.lg_bool,AeroIn_Bus.angleOfAttack_deg,AeroIn_Bus.angleOfSideslip_deg
  Crmblg_ : Subsystem
  Crmblg : Outport
  wires:
  Bus Selector/3 -> Crmblg_/3(angleOfSideslip_deg)  "<angleOfSideslip_deg>"
  Bus Selector/2 -> Crmblg_/2(angleOfAttack_deg)  "<angleOfAttack_deg>"
  Bus Selector/1 -> Crmblg_/1(dLG)  "<lg_bool>"
  in_bus/1 -> Bus Selector/1  "in_bus"
  Crmblg_/1(Crmblg) -> Crmblg/1

== system aerotest/RollMomentCoefficient/MachRegion3/Crmdai ==
  in_bus : Inport
  Bus Selector : BusSelector  OutputSignals=AeroIn_Bus.angleOfAttack_deg,AeroIn_Bus.dAI,AeroIn_Bus.mach_nd,AeroIn_Bus.dEI,eieff,AeroIn_Bus.qacorr
  Crmdai_ : Subsystem
  Crmdai : Outport
  wires:
  Bus Selector/6 -> Crmdai_/6(qacorr)  "<qacorr>"
  Bus Selector/5 -> Crmdai_/5(eieff)  "<eieff>"
  Bus Selector/4 -> Crmdai_/4(dEI)  "<dEI>"
  Bus Selector/3 -> Crmdai_/3(mach_nd)  "<mach_nd>"
  Bus Selector/2 -> Crmdai_/2(dAI)  "<dAI>"
  Bus Selector/1 -> Crmdai_/1(angleOfAttack_deg)  "<angleOfAttack_deg>"
  in_bus/1 -> Bus Selector/1  "in_bus"
  Crmdai_/1(Crmdai) -> Crmdai/1

== system aerotest/RollMomentCoefficient/MachRegion3/Crmdaib ==
  Constant : Constant  Value=0
  Crmdaib : Outport
  wires:
  Constant/1 -> Crmdaib/1

== system aerotest/RollMomentCoefficient/MachRegion3/Crmday ==
  in_bus : Inport
  Bus Selector : BusSelector  OutputSignals=AeroIn_Bus.angleOfAttack_deg,AeroIn_Bus.dAY,AeroIn_Bus.mach_nd,AeroIn_Bus.dEY,eoeff,AeroIn_Bus.qacorr
  Crmday_ : Subsystem
  Crmday : Outport
  wires:
  Bus Selector/1 -> Crmday_/1(angleOfAttack_deg)  "<angleOfAttack_deg>"
  Bus Selector/2 -> Crmday_/2(dAI)  "<dAY>"
  Bus Selector/3 -> Crmday_/3(mach_nd)  "<mach_nd>"
  Bus Selector/4 -> Crmday_/4(dEI)  "<dEY>"
  Bus Selector/5 -> Crmday_/5(eieff)  "<eoeff>"
  Bus Selector/6 -> Crmday_/6(qacorr)  "<qacorr>"
  Crmday_/1(Crmdai) -> Crmday/1
  in_bus/1 -> Bus Selector/1  "in_bus"

== system aerotest/RollMomentCoefficient/MachRegion3/Crmdayb ==
  Constant : Constant  Value=0
  Crmdayb : Outport
  wires:
  Constant/1 -> Crmdayb/1

== system aerotest/RollMomentCoefficient/MachRegion3/Crmdna ==
  in_bus : Inport
  Bus Selector : BusSelector  OutputSignals=AeroIn_Bus.angleOfAttack_deg,AeroIn_Bus.dNA
  Crmdna_ : Subsystem
  Crmdna : Outport
  wires:
  Bus Selector/2 -> Crmdna_/2(dNA)  "<dNA>"
  Bus Selector/1 -> Crmdna_/1(angleOfAttack_deg)  "<angleOfAttack_deg>"
  Crmdna_/1(Crmdna) -> Crmdna/1
  in_bus/1 -> Bus Selector/1  "in_bus"

== system aerotest/RollMomentCoefficient/MachRegion3/Crmdr ==
  in_bus : Inport
  Bus Selector : BusSelector  OutputSignals=AeroIn_Bus.qacorr,AeroIn_Bus.mach_nd,AeroIn_Bus.rud_deg
  Crmdr_ : Subsystem
  Crmdr : Outport
  wires:
  Bus Selector/3 -> Crmdr_/3(dR)  "<rud_deg>"
  Bus Selector/2 -> Crmdr_/2(mach_nd)  "<mach_nd>"
  Bus Selector/1 -> Crmdr_/1(qacorr)  "<qacorr>"
  Crmdr_/1(Crmdr) -> Crmdr/1
  in_bus/1 -> Bus Selector/1  "in_bus"

== system aerotest/RollMomentCoefficient/MachRegion3/Crmp ==
  in_bus : Inport
  Bus Selector : BusSelector  OutputSignals=AeroIn_Bus.angleOfAttack_deg,AeroIn_Bus.mach_nd,AeroIn_Bus.pc,AeroIn_Bus.qacorr
  Crmp_ : Subsystem
  Crmp : Outport
  wires:
  Bus Selector/4 -> Crmp_/4(qacorr)  "<qacorr>"
  Bus Selector/3 -> Crmp_/3(pc)  "<pc>"
  Bus Selector/2 -> Crmp_/2(mach_nd)  "<mach_nd>"
  Bus Selector/1 -> Crmp_/1(angleOfAttack_deg)  "<angleOfAttack_deg>"
  Crmp_/1(Crmp) -> Crmp/1
  in_bus/1 -> Bus Selector/1  "in_bus"

== system aerotest/RollMomentCoefficient/MachRegion3/Crmpbeta ==
  Crmpbeta_ : Constant  Value=0
  Crmpbeta : Outport
  wires:
  Crmpbeta_/1 -> Crmpbeta/1

== system aerotest/RollMomentCoefficient/MachRegion3/Crmr ==
  in_bus : Inport
  Bus Selector : BusSelector  OutputSignals=AeroIn_Bus.angleOfAttack_deg,AeroIn_Bus.mach_nd,AeroIn_Bus.rc
  Crmr_ : Subsystem
  Crmr : Outport
  wires:
  Bus Selector/3 -> Crmr_/3(rc)  "<rc>"
  Bus Selector/2 -> Crmr_/2(mach_nd)  "<mach_nd>"
  Bus Selector/1 -> Crmr_/1(angleOfAttack_deg)  "<angleOfAttack_deg>"
  Crmr_/1(Crmr) -> Crmr/1
  in_bus/1 -> Bus Selector/1  "in_bus"

== system aerotest/RollMomentCoefficient/MachRegion3/Crmrbeta ==
  Crmrbeta_ : Constant  Value=0
  Crmrbeta : Outport
  wires:
  Crmrbeta_/1 -> Crmrbeta/1

== system aerotest/RollMomentCoefficient/MachRegion3/Crmrde ==
  in_bus : Inport
  Bus Selector : BusSelector  OutputSignals=AeroIn_Bus.mach_nd,AeroIn_Bus.angleOfAttack_deg,AeroIn_Bus.rc,AeroIn_Bus.dEI,eieff,AeroIn_Bus.dEY,eoeff
  Crmrde_ : Subsystem
  Crmrde : Outport
  wires:
  Bus Selector/1 -> Crmrde_/1(mach_nd)  "<mach_nd>"
  Bus Selector/2 -> Crmrde_/2(angleOfAttack_deg)  "<angleOfAttack_deg>"
  Bus Selector/3 -> Crmrde_/3(rc)  "<rc>"
  Bus Selector/4 -> Crmrde_/4(dEI)  "<dEI>"
  Bus Selector/5 -> Crmrde_/5(eieff)  "<eieff>"
  Bus Selector/6 -> Crmrde_/6(dEY)  "<dEY>"
  Bus Selector/7 -> Crmrde_/7(eoeff)  "<eoeff>"
  Crmrde_/1(Crmrde) -> Crmrde/1
  in_bus/1 -> Bus Selector/1  "in_bus"

== system aerotest/RollMomentCoefficient/MachRegion3/eoeff1 ==
  AeroIn_Bus : Inport
  Bus Selector : BusSelector  OutputSignals=mach_nd
  CRMDAYOD_M : Lookup_n-D  NumberOfTableDimensions=1  BreakpointsForDimension1=admireDB.aerodata_asym_ext.CRMDAYOD.breakpoints.M  BreakpointsForDimension3=[5, 7]  Table=admireDB.aerodata_asym_ext.CRMDAYOD.newTable  ExtrapMethod=Clip  InternalRulePriority=Speed  RndMeth=Simplest  InputSameDT=on
  Constant : Constant
  Sum : Sum  Inputs=-+|
  eoeff : Outport
  eieff : Outport  Port=2
  wires:
  Sum/1 -> eieff/1
  CRMDAYOD_M/1 -> eoeff/1, Sum/1
  Constant/1 -> Sum/2
  Bus Selector/1 -> CRMDAYOD_M/1  "<mach_nd>"
  AeroIn_Bus/1 -> Bus Selector/1

== system aerotest/RollMomentCoefficient/MachRegion4/Crmbasic ==
  Constant : Constant  Value=0
  Crmbasic : Outport
  wires:
  Constant/1 -> Crmbasic/1

== system aerotest/RollMomentCoefficient/MachRegion4/Crmbde ==
  in_bus : Inport
  Bus Selector : BusSelector  OutputSignals=AeroIn_Bus.angleOfAttack_deg,AeroIn_Bus.dN,AeroIn_Bus.dEI,AeroIn_Bus.angleOfSideslip_deg,AeroIn_Bus.dEY,eieff,eoeff,AeroIn_Bus.mach_nd
  Crmbde_ : Subsystem
  Crmbde : Outport
  wires:
  Bus Selector/8 -> Crmbde_/8(mach_nd)  "<mach_nd>"
  Bus Selector/7 -> Crmbde_/7(eoeff)  "<eoeff>"
  Bus Selector/6 -> Crmbde_/6(eieff)  "<eieff>"
  Bus Selector/5 -> Crmbde_/5(dEY)  "<dEY>"
  Bus Selector/4 -> Crmbde_/4(angleOfSideslip_deg)  "<angleOfSideslip_deg>"
  Bus Selector/3 -> Crmbde_/3(dEI)  "<dEI>"
  Bus Selector/2 -> Crmbde_/2(dN)  "<dN>"
  Bus Selector/1 -> Crmbde_/1(angleOfAttack_deg)  "<angleOfAttack_deg>"
  Crmbde_/1(Crmbde) -> Crmbde/1
  in_bus/1 -> Bus Selector/1  "in_bus"

== system aerotest/RollMomentCoefficient/MachRegion4/Crmbdle ==
  in_bus : Inport
  Bus Selector : BusSelector  OutputSignals=AeroIn_Bus.angleOfAttack_deg,AeroIn_Bus.dEI,AeroIn_Bus.mach_nd,AeroIn_Bus.dEY,eieff,eoeff,AeroIn_Bus.angleOfSideslip_deg,AeroIn_Bus.lef_deg
  Crmbdle_ : Subsystem
  Crmbdle : Outport
  wires:
  Bus Selector/1 -> Crmbdle_/1(angleOfAttack_deg)  "<angleOfAttack_deg>"
  Bus Selector/2 -> Crmbdle_/2(dEI)  "<dEI>"
  Bus Selector/3 -> Crmbdle_/3(mach_nd)  "<mach_nd>"
  Bus Selector/4 -> Crmbdle_/4(dEY)  "<dEY>"
  Bus Selector/5 -> Crmbdle_/5(eieff)  "<eieff>"
  Bus Selector/6 -> Crmbdle_/6(eoeff)  "<eoeff>"
  Bus Selector/7 -> Crmbdle_/7(angleOfSideslip_deg)  "<angleOfSideslip_deg>"
  Bus Selector/8 -> Crmbdle_/8(dLE)  "<lef_deg>"
  Crmbdle_/1(Crmbdle) -> Crmbdle/1
  in_bus/1 -> Bus Selector/1  "in_bus"

== system aerotest/RollMomentCoefficient/MachRegion4/Crmbdn ==
  in_bus : Inport
  Bus Selector : BusSelector  OutputSignals=AeroIn_Bus.dN,AeroIn_Bus.mach_nd,AeroIn_Bus.angleOfSideslip_deg
  Crmbdn_ : Subsystem
  Crmbdn : Outport
  wires:
  Bus Selector/3 -> Crmbdn_/3(angleOfSideslip_deg)  "<angleOfSideslip_deg>"
  Bus Selector/1 -> Crmbdn_/1(dN)  "<dN>"
  Bus Selector/2 -> Crmbdn_/2(mach_nd)  "<mach_nd>"
  in_bus/1 -> Bus Selector/1  "in_bus"
  Crmbdn_/1(Crmbdn) -> Crmbdn/1

== system aerotest/RollMomentCoefficient/MachRegion4/Crmbeta ==
  in_bus : Inport
  Bus Selector : BusSelector  OutputSignals=AeroIn_Bus.mach_nd,AeroIn_Bus.angleOfAttack_deg,AeroIn_Bus.angleOfSideslip_deg,AeroIn_Bus.qacorr
  Crmbeta_ : Subsystem
  Crmbeta : Outport
  wires:
  Bus Selector/2 -> Crmbeta_/2(angleOfAttack_deg)  "<angleOfAttack_deg>"
  Bus Selector/1 -> Crmbeta_/1(mach_nd)  "<mach_nd>"
  Bus Selector/3 -> Crmbeta_/3(angleOfSideslip_deg)  "<angleOfSideslip_deg>"
  Bus Selector/4 -> Crmbeta_/4(qacorr)  "<qacorr>"
  in_bus/1 -> Bus Selector/1  "in_bus"
  Crmbeta_/1(Crmbeta) -> Crmbeta/1

== system aerotest/RollMomentCoefficient/MachRegion4/Crmbetad ==
  in_bus : Inport
  Bus Selector : BusSelector  OutputSignals=AeroIn_Bus.angleOfAttack_deg,AeroIn_Bus.mach_nd,AeroIn_Bus.betad
  Crmbetad_ : Subsystem
  Crmbetad : Outport
  wires:
  Bus Selector/3 -> Crmbetad_/3(betad)  "<betad>"
  Bus Selector/1 -> Crmbetad_/1(angleOfAttack_deg)  "<angleOfAttack_deg>"
  Bus Selector/2 -> Crmbetad_/2(mach_nd)  "<mach_nd>"
  in_bus/1 -> Bus Selector/1  "in_bus"
  Crmbetad_/1(Crmbetad) -> Crmbetad/1

== system aerotest/RollMomentCoefficient/MachRegion4/Crmblg ==
  in_bus : Inport
  Bus Selector : BusSelector  OutputSignals=AeroIn_Bus.lg_bool,AeroIn_Bus.angleOfAttack_deg,AeroIn_Bus.angleOfSideslip_deg
  Crmblg_ : Subsystem
  Crmblg : Outport
  wires:
  Bus Selector/3 -> Crmblg_/3(angleOfSideslip_deg)  "<angleOfSideslip_deg>"
  Bus Selector/2 -> Crmblg_/2(angleOfAttack_deg)  "<angleOfAttack_deg>"
  Bus Selector/1 -> Crmblg_/1(dLG)  "<lg_bool>"
  in_bus/1 -> Bus Selector/1  "in_bus"
  Crmblg_/1(Crmblg) -> Crmblg/1

== system aerotest/RollMomentCoefficient/MachRegion4/Crmdai ==
  in_bus : Inport
  Bus Selector : BusSelector  OutputSignals=AeroIn_Bus.angleOfAttack_deg,AeroIn_Bus.dEI,AeroIn_Bus.mach_nd,AeroIn_Bus.dAI,eieff,AeroIn_Bus.qacorr
  Crmdai_ : Subsystem
  Crmdai : Outport
  wires:
  Bus Selector/6 -> Crmdai_/6(qacorr)  "<qacorr>"
  Bus Selector/5 -> Crmdai_/5(eieff)  "<eieff>"
  Bus Selector/4 -> Crmdai_/4(dAI)  "<dAI>"
  Bus Selector/3 -> Crmdai_/3(mach_nd)  "<mach_nd>"
  Bus Selector/2 -> Crmdai_/2(dEI)  "<dEI>"
  Bus Selector/1 -> Crmdai_/1(angleOfAttack_deg)  "<angleOfAttack_deg>"
  in_bus/1 -> Bus Selector/1  "in_bus"
  Crmdai_/1(Crmdai) -> Crmdai/1

== system aerotest/RollMomentCoefficient/MachRegion4/Crmdaib ==
  Constant : Constant  Value=0
  Crmdaib : Outport
  wires:
  Constant/1 -> Crmdaib/1

== system aerotest/RollMomentCoefficient/MachRegion4/Crmday ==
  in_bus : Inport
  Bus Selector : BusSelector  OutputSignals=AeroIn_Bus.angleOfAttack_deg,AeroIn_Bus.dEY,AeroIn_Bus.mach_nd,AeroIn_Bus.dAY,eoeff,AeroIn_Bus.qacorr
  Crmday_ : Subsystem
  Crmday : Outport
  wires:
  Bus Selector/6 -> Crmday_/6(qacorr)  "<qacorr>"
  Bus Selector/5 -> Crmday_/5(eoeff)  "<eoeff>"
  Bus Selector/4 -> Crmday_/4(dAY)  "<dAY>"
  Bus Selector/3 -> Crmday_/3(mach_nd)  "<mach_nd>"
  Bus Selector/2 -> Crmday_/2(dEY)  "<dEY>"
  Bus Selector/1 -> Crmday_/1(angleOfAttack_deg)  "<angleOfAttack_deg>"
  Crmday_/1(Crmday) -> Crmday/1
  in_bus/1 -> Bus Selector/1  "in_bus"

== system aerotest/RollMomentCoefficient/MachRegion4/Crmdayb ==
  Constant : Constant  Value=0
  Crmdayb : Outport
  wires:
  Constant/1 -> Crmdayb/1

== system aerotest/RollMomentCoefficient/MachRegion4/Crmdna ==
  in_bus : Inport
  Bus Selector : BusSelector  OutputSignals=AeroIn_Bus.angleOfAttack_deg,AeroIn_Bus.dNA
  Crmdna_ : Subsystem
  Crmdna : Outport
  wires:
  Bus Selector/2 -> Crmdna_/2(dNA)  "<dNA>"
  Bus Selector/1 -> Crmdna_/1(angleOfAttack_deg)  "<angleOfAttack_deg>"
  Crmdna_/1(Crmdna) -> Crmdna/1
  in_bus/1 -> Bus Selector/1  "in_bus"

== system aerotest/RollMomentCoefficient/MachRegion4/Crmdr ==
  in_bus : Inport
  Bus Selector : BusSelector  OutputSignals=AeroIn_Bus.qacorr,AeroIn_Bus.mach_nd,AeroIn_Bus.rud_deg
  Crmdr_ : Subsystem
  Crmdr : Outport
  wires:
  Bus Selector/3 -> Crmdr_/3(dR)  "<rud_deg>"
  Bus Selector/2 -> Crmdr_/2(mach_nd)  "<mach_nd>"
  Bus Selector/1 -> Crmdr_/1(qacorr)  "<qacorr>"
  Crmdr_/1(Crmdr) -> Crmdr/1
  in_bus/1 -> Bus Selector/1  "in_bus"

== system aerotest/RollMomentCoefficient/MachRegion4/Crmp ==
  in_bus : Inport
  Bus Selector : BusSelector  OutputSignals=AeroIn_Bus.angleOfAttack_deg,AeroIn_Bus.mach_nd,AeroIn_Bus.pc,AeroIn_Bus.qacorr
  Crmp_ : Subsystem
  Crmp : Outport
  wires:
  Bus Selector/4 -> Crmp_/4(qacorr)  "<qacorr>"
  Bus Selector/3 -> Crmp_/3(pc)  "<pc>"
  Bus Selector/2 -> Crmp_/2(mach_nd)  "<mach_nd>"
  Bus Selector/1 -> Crmp_/1(angleOfAttack_deg)  "<angleOfAttack_deg>"
  Crmp_/1(Crmp) -> Crmp/1
  in_bus/1 -> Bus Selector/1  "in_bus"

== system aerotest/RollMomentCoefficient/MachRegion4/Crmpbeta ==
  Crmpbeta_ : Constant  Value=0
  Crmpbeta : Outport
  wires:
  Crmpbeta_/1 -> Crmpbeta/1

== system aerotest/RollMomentCoefficient/MachRegion4/Crmr ==
  in_bus : Inport
  Bus Selector : BusSelector  OutputSignals=AeroIn_Bus.angleOfAttack_deg,AeroIn_Bus.mach_nd,AeroIn_Bus.rc
  Crmr_ : Subsystem
  Crmr : Outport
  wires:
  Bus Selector/3 -> Crmr_/3(rc)  "<rc>"
  Bus Selector/2 -> Crmr_/2(mach_nd)  "<mach_nd>"
  Bus Selector/1 -> Crmr_/1(angleOfAttack_deg)  "<angleOfAttack_deg>"
  Crmr_/1(Crmr) -> Crmr/1
  in_bus/1 -> Bus Selector/1  "in_bus"

== system aerotest/RollMomentCoefficient/MachRegion4/Crmrbeta ==
  Crmrbeta_ : Constant  Value=0
  Crmrbeta : Outport
  wires:
  Crmrbeta_/1 -> Crmrbeta/1

== system aerotest/RollMomentCoefficient/MachRegion4/Crmrde ==
  in_bus : Inport
  Bus Selector : BusSelector  OutputSignals=AeroIn_Bus.mach_nd,AeroIn_Bus.angleOfAttack_deg,AeroIn_Bus.rc,AeroIn_Bus.dEI,eieff,AeroIn_Bus.dEY,eoeff
  Crmrde_ : Subsystem
  Crmrde : Outport
  wires:
  Bus Selector/1 -> Crmrde_/1(mach_nd)  "<mach_nd>"
  Bus Selector/2 -> Crmrde_/2(angleOfAttack_deg)  "<angleOfAttack_deg>"
  Bus Selector/3 -> Crmrde_/3(rc)  "<rc>"
  Bus Selector/4 -> Crmrde_/4(dEI)  "<dEI>"
  Bus Selector/5 -> Crmrde_/5(eieff)  "<eieff>"
  Bus Selector/6 -> Crmrde_/6(dEY)  "<dEY>"
  Bus Selector/7 -> Crmrde_/7(eoeff)  "<eoeff>"
  Crmrde_/1(Crmrde) -> Crmrde/1
  in_bus/1 -> Bus Selector/1  "in_bus"

== system aerotest/RollMomentCoefficient/MachRegion4/eoeff1 ==
  AeroIn_Bus : Inport
  Bus Selector : BusSelector  OutputSignals=mach_nd
  CRMDAYOD_M : Lookup_n-D  NumberOfTableDimensions=1  BreakpointsForDimension1=admireDB.aerodata_asym_ext.CRMDAYOD.breakpoints.M  BreakpointsForDimension3=[5, 7]  Table=admireDB.aerodata_asym_ext.CRMDAYOD.newTable  ExtrapMethod=Clip  InternalRulePriority=Speed  RndMeth=Simplest  InputSameDT=on
  Constant : Constant
  Sum : Sum  Inputs=-+|
  eoeff : Outport
  eieff : Outport  Port=2
  wires:
  Sum/1 -> eieff/1
  CRMDAYOD_M/1 -> eoeff/1, Sum/1
  Constant/1 -> Sum/2
  Bus Selector/1 -> CRMDAYOD_M/1  "<mach_nd>"
  AeroIn_Bus/1 -> Bus Selector/1

== system aerotest/TangentialForceCoefficient/MachRegion1/Ctalfa ==
  in_bus : Inport
  Bus Selector : BusSelector  OutputSignals=AeroIn_Bus.angleOfAttack_deg
  CTAL_ALFA : Lookup_n-D  NumberOfTableDimensions=1  BreakpointsForDimension1=admireDB.aerodata_sym.CTAL.breakpoints.ALFA  BreakpointsForDimension3=[5, 7]  Table=admireDB.aerodata_sym.CTAL.newTable  ExtrapMethod=Clip  InternalRulePriority=Speed  RndMeth=Simplest  InputSameDT=on
  Ctalfa : Outport
  wires:
  Bus Selector/1 -> CTAL_ALFA/1  "<angleOfAttack_deg>"
  in_bus/1 -> Bus Selector/1
  CTAL_ALFA/1 -> Ctalfa/1  "Ctalfa"

== system aerotest/TangentialForceCoefficient/MachRegion1/Ctbasic ==
  in_bus : Inport
  Bus Selector : BusSelector  OutputSignals=AeroIn_Bus.mach_nd,AeroIn_Bus.altitude_m
  CTH_H_M : Lookup_n-D  BreakpointsForDimension1=admireDB.aerodata_sym.CTH.breakpoints.M  BreakpointsForDimension2=admireDB.aerodata_sym.CTH.breakpoints.H  BreakpointsForDimension3=[5, 7]  Table=admireDB.aerodata_sym.CTH.newTable  ExtrapMethod=Clip  InternalRulePriority=Speed  RndMeth=Simplest  InputSameDT=on
      settings: InputPortMap=u0,u1
  CTZERO_M : Lookup_n-D  NumberOfTableDimensions=1  BreakpointsForDimension1=admireDB.aerodata_sym.CTZERO.breakpoints.M  BreakpointsForDimension3=[5, 7]  Table=admireDB.aerodata_sym.CTZERO.newTable  ExtrapMethod=Clip  InternalRulePriority=Speed  RndMeth=Simplest  InputSameDT=on
  Constant : Constant  Value=1/1000
  Product : Product
  Sum1 : Sum  Inputs=|++
  Ctbasic : Outport
  wires:
  Sum1/1 -> Ctbasic/1
  CTZERO_M/1 -> Sum1/1
  CTH_H_M/1 -> Sum1/2
  Constant/1 -> Product/2
  Product/1 -> CTH_H_M/2
  Bus Selector/2 -> Product/1  "<altitude_m>"
  Bus Selector/1 -> CTZERO_M/1, CTH_H_M/1  "<mach_nd>"
  in_bus/1 -> Bus Selector/1  "in_bus"

== system aerotest/TangentialForceCoefficient/MachRegion1/Ctbeta ==
  in_bus : Inport
  Abs : Abs
  Bus Selector : BusSelector  OutputSignals=AeroIn_Bus.angleOfAttack_deg,AeroIn_Bus.dN,AeroIn_Bus.angleOfSideslip_deg
  CTBETA_DN_ALFA : Lookup_n-D  BreakpointsForDimension1=admireDB.aerodata_sym.CTBETA.breakpoints.ALFA  BreakpointsForDimension2=admireDB.aerodata_sym.CTBETA.breakpoints.DN  BreakpointsForDimension3=[5, 7]  Table=admireDB.aerodata_sym.CTBETA.newTable  ExtrapMethod=Clip  InternalRulePriority=Speed  RndMeth=Simplest  InputSameDT=on
      settings: InputPortMap=u0,u1
  CTKB_BETA : Lookup_n-D  NumberOfTableDimensions=1  BreakpointsForDimension1=admireDB.aerodata_sym.CTKB.breakpoints.BETA  BreakpointsForDimension3=[5, 7]  Table=admireDB.aerodata_sym.CTKB.newTable  ExtrapMethod=Clip  InternalRulePriority=Speed  RndMeth=Simplest  InputSameDT=on
  Product : Product
  Ctbeta : Outport
  wires:
  Product/1 -> Ctbeta/1
  CTBETA_DN_ALFA/1 -> Product/1
  CTKB_BETA/1 -> Product/2
  Abs/1 -> CTKB_BETA/1
  Bus Selector/3 -> Abs/1  "<angleOfSideslip_deg>"
  Bus Selector/1 -> CTBETA_DN_ALFA/1  "<angleOfAttack_deg>"
  Bus Selector/2 -> CTBETA_DN_ALFA/2  "<dN>"
  in_bus/1 -> Bus Selector/1

== system aerotest/TangentialForceCoefficient/MachRegion1/Ctda ==
  in_bus : Inport
  Abs : Abs
  Abs1 : Abs
  Abs2 : Abs
  Bus Selector : BusSelector  OutputSignals=AeroIn_Bus.angleOfAttack_deg,AeroIn_Bus.dAI,AeroIn_Bus.dAY
  Bus Selector1 : BusSelector  OutputSignals=eieff,eoeff
  CTDAAL_DA_ALFA : Lookup_n-D  BreakpointsForDimension1=admireDB.aerodata_sym.CTDAAL.breakpoints.ALFA  BreakpointsForDimension2=admireDB.aerodata_sym.CTDAAL.breakpoints.DA  BreakpointsForDimension3=[5, 7]  Table=admireDB.aerodata_sym.CTDAAL.newTable  ExtrapMethod=Clip  InternalRulePriority=Speed  RndMeth=Simplest  InputSameDT=on
      settings: InputPortMap=u0,u1
  CTDAAL_DA_ALFA1 : Lookup_n-D  BreakpointsForDimension1=admireDB.aerodata_sym.CTDAAL.breakpoints.ALFA  BreakpointsForDimension2=admireDB.aerodata_sym.CTDAAL.breakpoints.DA  BreakpointsForDimension3=[5, 7]  Table=admireDB.aerodata_sym.CTDAAL.newTable  ExtrapMethod=Clip  InternalRulePriority=Speed  RndMeth=Simplest  InputSameDT=on
      settings: InputPortMap=u0,u1
  Product : Product
  Product1 : Product
  Sum : Sum  Inputs=|++
  Ctda : Outport
  wires:
  Sum/1 -> Ctda/1
  Product1/1 -> Sum/2
  Product/1 -> Sum/1
  Bus Selector1/2 -> Product1/1  "<eoeff>"
  CTDAAL_DA_ALFA1/1 -> Product1/2
  Bus Selector1/1 -> Product/1  "<eieff>"
  CTDAAL_DA_ALFA/1 -> Product/2
  Abs2/1 -> CTDAAL_DA_ALFA1/2
  Abs1/1 -> CTDAAL_DA_ALFA/2
  Abs/1 -> CTDAAL_DA_ALFA/1, CTDAAL_DA_ALFA1/1
  Bus Selector/2 -> Abs1/1  "<dAI>"
  Bus Selector/1 -> Abs/1  "<angleOfAttack_deg>"
  in_bus/1 -> Bus Selector/1, Bus Selector1/1
  Bus Selector/3 -> Abs2/1  "<dAY>"

== system aerotest/TangentialForceCoefficient/MachRegion1/Ctdedn ==
  in_bus : Inport
  Bus Selector : BusSelector  OutputSignals=AeroIn_Bus.angleOfAttack_deg,AeroIn_Bus.dE,AeroIn_Bus.dN
  CTDNDE_ALFA_DE_DN : Lookup_n-D  NumberOfTableDimensions=3  BreakpointsForDimension1=admireDB.aerodata_sym.CTDNDE.breakpoints.ALFA  BreakpointsForDimension2=admireDB.aerodata_sym.CTDNDE.breakpoints.DE  BreakpointsForDimension3=admireDB.aerodata_sym.CTDNDE.breakpoints.DN  Table=admireDB.aerodata_sym.CTDNDE.newTable  ExtrapMethod=Clip  InternalRulePriority=Speed  RndMeth=Simplest  InputSameDT=on
      settings: InputPortMap=u0,u1,u2
  Ctdedn : Outport
  wires:
  Bus Selector/1 -> CTDNDE_ALFA_DE_DN/1  "<angleOfAttack_deg>"
  Bus Selector/3 -> CTDNDE_ALFA_DE_DN/3  "<dN>"
  CTDNDE_ALFA_DE_DN/1 -> Ctdedn/1
  Bus Selector/2 -> CTDNDE_ALFA_DE_DN/2  "<dE>"
  in_bus/1 -> Bus Selector/1

== system aerotest/TangentialForceCoefficient/MachRegion1/Ctdei ==
  in_bus : Inport
  Bus Selector : BusSelector  OutputSignals=AeroIn_Bus.angleOfAttack_deg,AeroIn_Bus.dEI,eieff
  CTDEAL_DE_ALFA : Lookup_n-D  BreakpointsForDimension1=admireDB.aerodata_sym.CTDEAL.breakpoints.ALFA  BreakpointsForDimension2=admireDB.aerodata_sym.CTDEAL.breakpoints.DE  BreakpointsForDimension3=[5, 7]  Table=admireDB.aerodata_sym.CTDEAL.newTable  ExtrapMethod=Clip  InternalRulePriority=Speed  RndMeth=Simplest  InputSameDT=on
      settings: InputPortMap=u0,u1
  Product : Product
  Ctdei : Outport
  wires:
  Product/1 -> Ctdei/1
  Bus Selector/3 -> Product/2  "<eieff>"
  CTDEAL_DE_ALFA/1 -> Product/1
  Bus Selector/1 -> CTDEAL_DE_ALFA/1  "<angleOfAttack_deg>"
  Bus Selector/2 -> CTDEAL_DE_ALFA/2  "<dEI>"
  in_bus/1 -> Bus Selector/1

== system aerotest/TangentialForceCoefficient/MachRegion1/Ctdey ==
  in_bus : Inport
  Bus Selector : BusSelector  OutputSignals=AeroIn_Bus.angleOfAttack_deg,AeroIn_Bus.dEY,eoeff
  CTDEAL_DE_ALFA : Lookup_n-D  BreakpointsForDimension1=admireDB.aerodata_sym.CTDEAL.breakpoints.ALFA  BreakpointsForDimension2=admireDB.aerodata_sym.CTDEAL.breakpoints.DE  BreakpointsForDimension3=[5, 7]  Table=admireDB.aerodata_sym.CTDEAL.newTable  ExtrapMethod=Clip  InternalRulePriority=Speed  RndMeth=Simplest  InputSameDT=on
      settings: InputPortMap=u0,u1
  Product : Product
  Ctdey : Outport
  wires:
  in_bus/1 -> Bus Selector/1
  Bus Selector/2 -> CTDEAL_DE_ALFA/2  "<dEY>"
  Bus Selector/1 -> CTDEAL_DE_ALFA/1  "<angleOfAttack_deg>"
  CTDEAL_DE_ALFA/1 -> Product/1
  Bus Selector/3 -> Product/2  "<eoeff>"
  Product/1 -> Ctdey/1

== system aerotest/TangentialForceCoefficient/MachRegion1/Ctdle ==
  in_bus : Inport
  Bus Selector : BusSelector  OutputSignals=AeroIn_Bus.angleOfAttack_deg,AeroIn_Bus.lef_deg,AeroIn_Bus.dN
  CTDLEAL_DLE_ALFA : Lookup_n-D  BreakpointsForDimension1=admireDB.aerodata_sym.CTDLEAL.breakpoints.ALFA  BreakpointsForDimension2=admireDB.aerodata_sym.CTDLEAL.breakpoints.DLE  BreakpointsForDimension3=[5, 7]  Table=admireDB.aerodata_sym.CTDLEAL.newTable  ExtrapMethod=Clip  InternalRulePriority=Speed  RndMeth=Simplest  InputSameDT=on
      settings: InputPortMap=u0,u1
  CTLEDNAL_DN_ALFA : Lookup_n-D  BreakpointsForDimension1=admireDB.aerodata_sym.CTLEDNAL.breakpoints.ALFA  BreakpointsForDimension2=admireDB.aerodata_sym.CTLEDNAL.breakpoints.DN  BreakpointsForDimension3=[5, 7]  Table=admireDB.aerodata_sym.CTLEDNAL.newTable  ExtrapMethod=Clip  InternalRulePriority=Speed  RndMeth=Simplest  InputSameDT=on
      settings: InputPortMap=u0,u1
  Constant : Constant  Value=1/27
  Product : Product  Inputs=3
  Sum : Sum  Inputs=|++
  Ctdle : Outport
  wires:
  Product/1 -> Sum/2
  Constant/1 -> Product/3
  CTLEDNAL_DN_ALFA/1 -> Product/1
  Bus Selector/3 -> CTLEDNAL_DN_ALFA/2  "<dN>"
  Sum/1 -> Ctdle/1
  Bus Selector/1 -> CTLEDNAL_DN_ALFA/1, CTDLEAL_DLE_ALFA/1  "<angleOfAttack_deg>"
  Bus Selector/2 -> Product/2, CTDLEAL_DLE_ALFA/2  "<lef_deg>"
  CTDLEAL_DLE_ALFA/1 -> Sum/1
  in_bus/1 -> Bus Selector/1

== system aerotest/TangentialForceCoefficient/MachRegion1/Ctdn ==
  in_bus : Inport
  Bus Selector : BusSelector  OutputSignals=AeroIn_Bus.angleOfAttack_deg,AeroIn_Bus.dN
  CTDNAL_DN_ALFA : Lookup_n-D  BreakpointsForDimension1=admireDB.aerodata_sym.CTDNAL.breakpoints.ALFA  BreakpointsForDimension2=admireDB.aerodata_sym.CTDNAL.breakpoints.DN  BreakpointsForDimension3=[5, 7]  Table=admireDB.aerodata_sym.CTDNAL.newTable  ExtrapMethod=Clip  InternalRulePriority=Speed  RndMeth=Simplest  InputSameDT=on
      settings: InputPortMap=u0,u1
  Ctdn : Outport
  wires:
  in_bus/1 -> Bus Selector/1
  CTDNAL_DN_ALFA/1 -> Ctdn/1
  Bus Selector/2 -> CTDNAL_DN_ALFA/2  "<dN>"
  Bus Selector/1 -> CTDNAL_DN_ALFA/1  "<angleOfAttack_deg>"

== system aerotest/TangentialForceCoefficient/MachRegion1/Ctdr ==
  in_bus : Inport
  Abs : Abs
  Bus Selector : BusSelector  OutputSignals=AeroIn_Bus.mach_nd,AeroIn_Bus.rud_deg
  CTMDR_DR_M : Lookup_n-D  BreakpointsForDimension1=admireDB.aerodata_sym.CTMDR.breakpoints.M  BreakpointsForDimension2=admireDB.aerodata_sym.CTMDR.breakpoints.DR  BreakpointsForDimension3=[5, 7]  Table=admireDB.aerodata_sym.CTMDR.newTable  ExtrapMethod=Clip  InternalRulePriority=Speed  RndMeth=Simplest  InputSameDT=on
      settings: InputPortMap=u0,u1
  Ctdr : Outport
  wires:
  Abs/1 -> CTMDR_DR_M/2
  Bus Selector/1 -> CTMDR_DR_M/1  "<mach_nd>"
  Bus Selector/2 -> Abs/1  "<rud_deg>"
  in_bus/1 -> Bus Selector/1
  CTMDR_DR_M/1 -> Ctdr/1
